simulink model "car_16b"  (R2016b)
settings: Solver=ode3  StartTime=0.0  StopTime=4000  FixedStep=0.1  MaxStep=1e-4  RelTol=1e-3
values from neighbouring files (symbols this model uses):
  A = 2.2    [constant.m]
  alpha = 0    [constant.m]
  C_D = 0.35    [constant.m]
  C_e = 4.4    [constant.m]
  C_t = 42    [constant.m]
  f = 0.018    [constant.m]
  g = 9.8    [constant.m]
  i_g = 2    [constant.m]
  J_m = 0.25    [constant.m]
  J_w = 4    [constant.m]
  K_p = 4    [constant.m]
  m = 1000    [constant.m]
  Phi = 0.028    [constant.m]
  r_w = 0.28    [constant.m]
  Ra = 0.088    [constant.m]
  rou = 1.226    [constant.m]
  T_i = 1    [constant.m]
  yita = 0.8    [constant.m]
undefined symbols (not defined in the file or in its folder): Ion, Lithium, sgn
libraries: electricdrivelib x5, powerlib x3, simulink x1
settings Model: Creator=Dorian  LastModifiedBy=Dorian
settings DataIOCC: SaveCompleteFinalSimState=on  SaveFormat=StructureWithTime  SaveOutput=off  ReturnWorkspaceOutputs=on  LoggingToFile=on
settings OptimizationCC: PassReuseOutputArgsThreshold=0
settings DebuggingCC: ParameterTunabilityLossMsg=error
settings RTWCC: PackageName=car_test  TemplateMakefile=RTW.MSVCBuild  Description=Create Visual C/C++ Solution File for Simulink Coder  GenerateReport=on  RTWVerbose=off  LaunchReport=on  TargetLang=C++  RTWCompilerOptimization=on
settings CodeAppCC: ForceParamTrailComments=on  OperatorAnnotations=on
settings GRTTargetCC: TargetLangStandard=C++03 (ISO)  MultiInstanceERTCode=on  CodeInterfacePackaging=C++ class
settings SimscapeCC: SimscapeUseOperatingPoints=on  SimscapeOperatingPoint=u

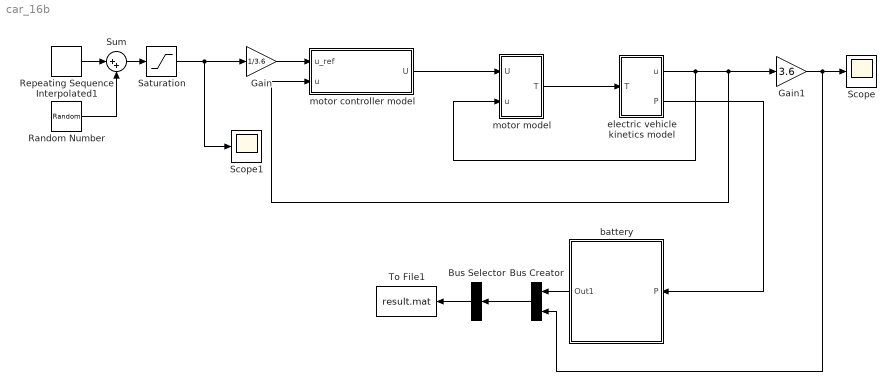
== system car_16b ==
  Bus Creator : BusCreator  Inputs=2
  Bus Selector : BusSelector  OutputSignals=signal1.SOC (%),signal1.Cell Temperature (oC),signal1.Current (A),signal1.Voltage (V),signal2  OutputAsBus=on
  Gain : Gain  Gain=1/3.6
  Gain1 : Gain  Gain=3.6
  Random Number : RandomNumber  SampleTime=1
  Repeating Sequence Interpolated1 : simulink/Sources/Repeating Sequence Interpolated  OutValues=y  TimeValues=x  LookUpMeth=Use Input Above  tsamp=0.1  OutMin=[]  OutMax=[]  OutDataTypeStr=double  OutputDataTypeScalingMode=double  OutDataType=fixdt(0,8)  OutScaling=2^-10
  Saturation : Saturate  UpperLimit=inf  LowerLimit=0
  Scope : Scope
  Scope1 : Scope
  Sum : Sum  Inputs=|++
  To File1 : ToFile  Filename=result.mat
  battery : Subsystem
  electric vehicle kinetics model : Subsystem
  motor controller model : Subsystem
  motor model : Subsystem
  wires:
  motor model/1(T) -> electric vehicle kinetics model/1(T)
  electric vehicle kinetics model/1(u) -> motor model/2(u), motor controller model/2(u), Gain1/1
  motor controller model/1(U) -> motor model/1(U)
  electric vehicle kinetics model/2(P) -> battery/1(P)
  Gain/1 -> motor controller model/1(u_ref)
  Gain1/1 -> Bus Creator/2, Scope/1
  Sum/1 -> Saturation/1
  Random Number/1 -> Sum/2
  Saturation/1 -> Scope1/1, Gain/1
  Repeating Sequence Interpolated1/1 -> Sum/1
  battery/1(Out1) -> Bus Creator/1
  Bus Selector/1 -> To File1/1
  Bus Creator/1 -> Bus Selector/1

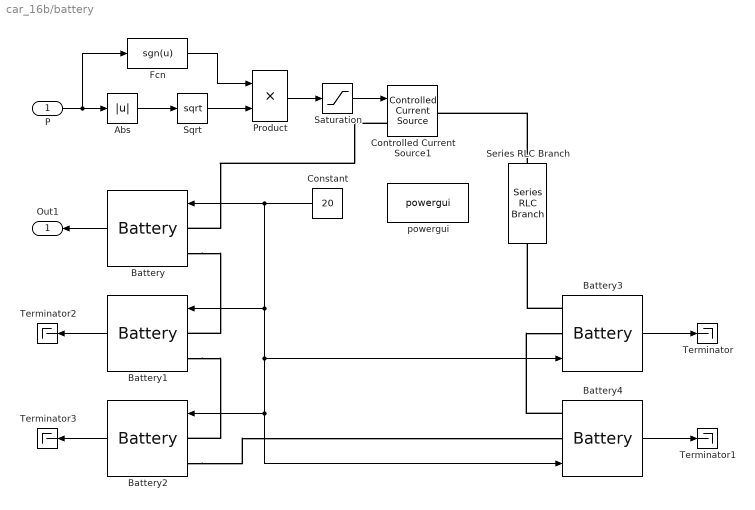
== system car_16b/battery ==
  P : Inport
  Abs : Abs
  Battery{,1..4} (5 alike) : electricdrivelib/Extra Sources/Battery  BatType=Lithium-Ion  ShowTempParam=on  ThermalPreset="12.8V  40Ah  (LiFeMgPO4)"  ShowAgeParam=on  NomV=12.6  NomQ=40  SOC=100  Batt_Tr=30  PresetModel=off  MaxQ=40  MinV=10.5  FullV=13.8  Dis_rate=20  R=0.015  Normal_OP=30.14  expZone="[13.1          0.5]"  current=[6.5 13 32.5]  Units=Time  Tci=20  NomT=20  T2=0  MaxQ2=36  FullV2=13  Normal_OP2=11.7  expZone2="[12.67            4]"  Rca=0.6411  ti=4880  Dp=0  Neq0=0  Tsim=1e6  Ta1=25  Qeol=5.4*0.9  Reol=0.013333*1.2  Char_age=[2.3478, 3]  Dis_age=[2.3478, 10]  N1=1500  N2=10500  N3=1000  N4=1400  Ta2=45  N5=950
  Constant : Constant  Value=20
  Controlled Current Source1 : powerlib/Electrical Sources/Controlled Current Source  Initialize=on  Source_Type=AC  Amplitude=0  Phase=0  Frequency=0  Measurements=None
  Fcn : Fcn  Expr=sgn(u)
  Product : Product
  Saturation : Saturate  UpperLimit=inf  LowerLimit=-20
  Series RLC Branch : powerlib/Elements/Series RLC Branch  LConnTagsString=__new0  RConnTagsString=__new0  BranchType=RLC  Resistance=1  Inductance=0  SetiL0=off  InitialCurrent=0  Capacitance=inf  Setx0=off  InitialVoltage=0  Measurements=None
  Sqrt : Sqrt  SaturateOnIntegerOverflow=on
  Terminator{,1..3} (4 alike) : Terminator
  powergui : powerlib/powergui  Priority=1  SimulationMode=Discrete  SampleTime=0.1  frequency=60  Iterations=50  frequencyindice=0  Pbase=100e6  ErrMax=1e-4  UnitsV=kV  UnitsW=MW  buscounter=0  FunctionMessages=off  echomessages=off  EnableUseOfTLC=off  CurrentSourceSwitches=off  DisableSnubberDevices=off  DisableRonSwitches=off  DisableVfSwitches=off  DisplayEquations=off  SolverType=Tustin/Backward Euler (TBE)  Interpol=off  ExternalGateDelay=off  methode=off  Ts=100  x0status=blocks  SPID=off  SwTol=0  HookPort=off  RestoreLinks=warning  ResistiveCurrentMeasurement=off  Frange=[0:2:500]  Ylog=off  Xlog=on  ShowGrid=off  save=off  variable=ZData  structure=0  ZoomFFT=off  StartTime=0.0  cycles=1  DisplayStyle=1  fundamental=60  FreqAxis=off  MaxFrequency=1000  frequencyindicesteady=1  RmsSteady=1  display=off
  Out1 : Outport
  wires:
  Constant/1 -> Battery3/1, Battery4/1, Battery2/1, Battery1/1, Battery/1
  Battery/1 -> Out1/1
  Battery1/1 -> Terminator2/1
  Battery3/1 -> Terminator/1
  Battery4/1 -> Terminator1/1
  Battery2/1 -> Terminator3/1
  Abs/1 -> Sqrt/1
  Product/1 -> Saturation/1
  Sqrt/1 -> Product/2
  P/1 -> Abs/1, Fcn/1
  Fcn/1 -> Product/1
  Saturation/1 -> Controlled Current Source1/1
  connections:
  Series RLC Branch/LConn1 -- Controlled Current Source1/RConn1
  Controlled Current Source1/LConn1 -- Battery/LConn1
  Battery/LConn2 -- Battery1/LConn1
  Battery1/LConn2 -- Battery2/LConn1
  Battery2/LConn2 -- Battery4/LConn1
  Battery4/LConn2 -- Battery3/LConn1
  Battery3/LConn2 -- Series RLC Branch/RConn1

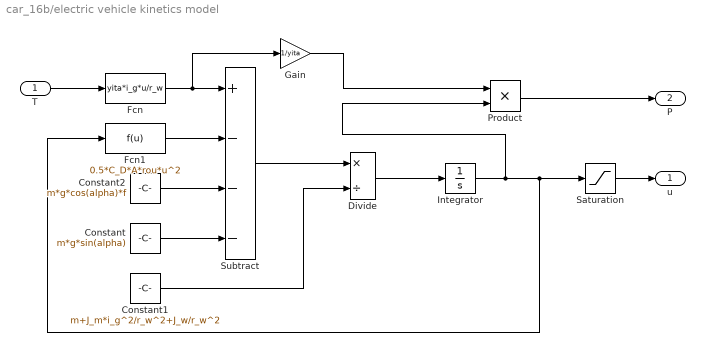
== system car_16b/electric vehicle kinetics model ==
  T : Inport
  Constant : Constant  Value=m*g*sin(alpha)
  Constant1 : Constant  Value=m+J_m*i_g^2/r_w^2+J_w/r_w^2
  Constant2 : Constant  Value=m*g*cos(alpha)*f
  Divide : Product  Inputs=*/
  Fcn : Fcn  Expr=yita*i_g*u/r_w
  Fcn1 : Fcn  Expr=0.5*C_D*A*rou*u^2
  Gain : Gain  Gain=1/yita
  Integrator : Integrator
  Product : Product
  Saturation : Saturate  UpperLimit=inf  LowerLimit=0
  Subtract : Sum  Inputs=+---
  u : Outport
  P : Outport  Port=2
  wires:
  T/1 -> Fcn/1
  Constant/1 -> Subtract/4
  Subtract/1 -> Divide/1
  Constant1/1 -> Divide/2
  Divide/1 -> Integrator/1
  Constant2/1 -> Subtract/3
  Fcn1/1 -> Subtract/2
  Product/1 -> P/1
  Fcn/1 -> Gain/1, Subtract/1
  Gain/1 -> Product/1
  Integrator/1 -> Saturation/1, Fcn1/1, Product/2
  Saturation/1 -> u/1

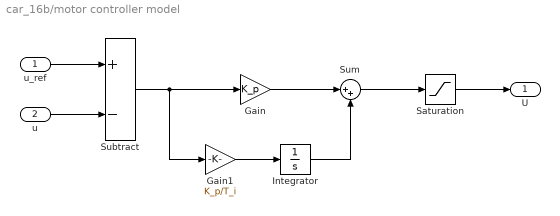
== system car_16b/motor controller model ==
  u_ref : Inport
  u : Inport  Port=2
  Gain : Gain  Gain=K_p
  Gain1 : Gain  Gain=K_p/T_i
  Integrator : Integrator
  Saturation : Saturate  UpperLimit=336  LowerLimit=-336
  Subtract : Sum  Inputs=+-
  Sum : Sum  Inputs=|++
  U : Outport
  wires:
  u/1 -> Subtract/2
  u_ref/1 -> Subtract/1
  Subtract/1 -> Gain1/1, Gain/1
  Gain/1 -> Sum/1
  Integrator/1 -> Sum/2
  Gain1/1 -> Integrator/1
  Sum/1 -> Saturation/1
  Saturation/1 -> U/1

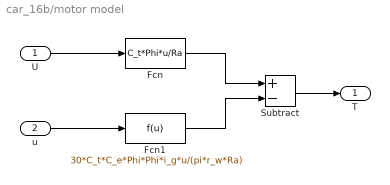
== system car_16b/motor model ==
  U : Inport
  u : Inport  Port=2
  Fcn : Fcn  Expr=C_t*Phi*u/Ra
  Fcn1 : Fcn  Expr=30*C_t*C_e*Phi*Phi*i_g*u/(pi*r_w*Ra)
  Subtract : Sum  Inputs=+-
  T : Outport
  wires:
  U/1 -> Fcn/1
  Fcn/1 -> Subtract/1
  Fcn1/1 -> Subtract/2
  u/1 -> Fcn1/1
  Subtract/1 -> T/1
